simulink model "S3"  (R2023b)
settings: Solver=FixedStepAuto  StartTime=0.0  StopTime=Time  FixedStep=Step_T  RelTol=1e-3
values from neighbouring files (symbols this model uses):
  x_1_0 = 2    [P_sim.m]
  x_2_0 = -2    [P_sim.m]
undefined symbols (not defined in the file or in its folder): alpha_1_d_0
settings Model: Creator=admin  LastModifiedBy=admin

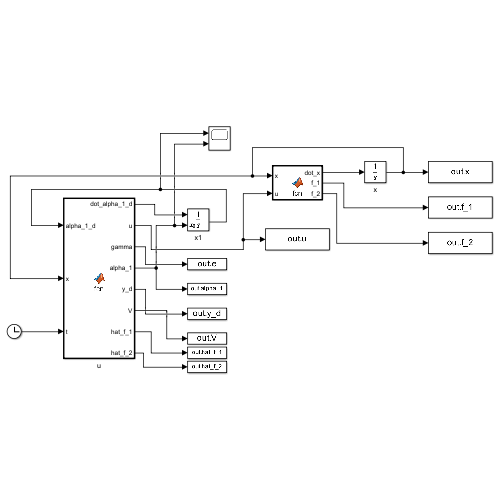
[thumbnail: Simulink's stored preview of the top-level diagram]
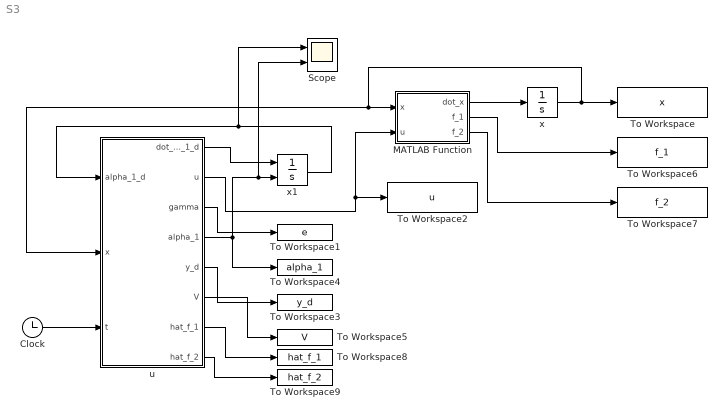
== system S3 ==
  Clock : Clock
  MATLAB Function : MATLAB Function  TreatAsAtomicUnit=on
  Scope : Scope  NumInputPorts=2
  To Workspace : ToWorkspace  VariableName=x  SaveFormat=Timeseries  SampleTime=-1
  To Workspace1 : ToWorkspace  VariableName=e  SaveFormat=Timeseries  SampleTime=-1
  To Workspace2 : ToWorkspace  VariableName=u  SaveFormat=Timeseries  SampleTime=-1
  To Workspace3 : ToWorkspace  VariableName=y_d  SaveFormat=Timeseries  SampleTime=-1
  To Workspace4 : ToWorkspace  VariableName=alpha_1  SaveFormat=Timeseries  SampleTime=-1
  To Workspace5 : ToWorkspace  VariableName=V  SaveFormat=Timeseries  SampleTime=-1
  To Workspace6 : ToWorkspace  VariableName=f_1  SaveFormat=Timeseries  SampleTime=-1
  To Workspace7 : ToWorkspace  VariableName=f_2  SaveFormat=Timeseries  SampleTime=-1
  To Workspace8 : ToWorkspace  VariableName=hat_f_1  SaveFormat=Timeseries  SampleTime=-1
  To Workspace9 : ToWorkspace  VariableName=hat_f_2  SaveFormat=Timeseries  SampleTime=-1
  u : MATLAB Function  TreatAsAtomicUnit=on
  x : Integrator  InitialCondition=[x_1_0;x_2_0]
  x1 : Integrator  InitialConditionSource=external  InitialCondition=alpha_1_d_0
  wires:
  MATLAB Function/1(dot_x) -> x/1
  x/1 -> To Workspace/1, u/2(x), MATLAB Function/1(x)
  u/2(u) -> MATLAB Function/2(u), To Workspace2/1
  u/3(gamma) -> To Workspace1/1
  u/5(y_d) -> To Workspace3/1
  Clock/1 -> u/3(t)
  u/1(dot_alpha_1_d) -> x1/1
  x1/1 -> Scope/1, u/1(alpha_1_d)
  u/4(alpha_1) -> To Workspace4/1, Scope/2, x1/2
  u/6(V) -> To Workspace5/1
  MATLAB Function/2(f_1) -> To Workspace6/1
  MATLAB Function/3(f_2) -> To Workspace7/1
  u/7(hat_f_1) -> To Workspace8/1
  u/8(hat_f_2) -> To Workspace9/1

== matlab function S3/u ==
  data: alpha_1_d input; dot_alpha_1_d output; x input; t input; u output; gamma output; alpha_1 output; pam parameter; y_d output; V output; hat_f_1 output; hat_f_2 output
function [dot_alpha_1_d,u,gamma,alpha_1,y_d,V,hat_f_1,hat_f_2]  = fcn(alpha_1_d,x,t,pam)

y_d = 5*sin(t);
dot_y_d = 5*cos(t);

x_1 = x(1);
x_2 = x(2);

z_1 = [sin(x_1);cos(x_1)];
z_2 = [sin(x_1);sin(x_2)];

%% 第一阶
e_1 = x_1 - y_d;
alpha_1 = -pam.lambda_1*e_1-pam.hat_theta_1'*z_1+dot_y_d;
 
%% 第二阶
e_2 = x_2 - alpha_1;
dot_alpha_1_d = -(1/pam.omega_1)*(alpha_1_d-alpha_1);
u = -pam.lambda_2*e_2-pam.hat_theta_2'*z_2+dot_alpha_1_d;
e_alpha_1 = alpha_1_d-alpha_1;

gamma = [e_1;e_2;e_alpha_1];

V = norm(gamma);

hat_f_1 = pam.hat_theta_1'*z_1;
hat_f_2 = pam.hat_theta_2'*z_2;

== matlab function S3/MATLAB Function ==
  data: x input; dot_x output; u input; f_1 output; f_2 output
function [dot_x,f_1,f_2]  = fcn(x,u)

x_1 = x(1);
x_2 = x(2);

f_1 = -2*sin(x_1)+3*cos(x_1);
f_2 = -0.5*sin(x_1)+2*sin(x_2);

dot_x_1 = x_2+f_1;
dot_x_2 = u+f_2;

dot_x = [dot_x_1;dot_x_2];
